simulink model "lab4_simulink3model2"  (R2024a)
settings: Solver=VariableStepAuto  StartTime=0.0  StopTime=1  RelTol=1e-3
libraries: commanabbnd3 x2
settings Model: Creator=PULLEY  LastModifiedBy=PULLEY

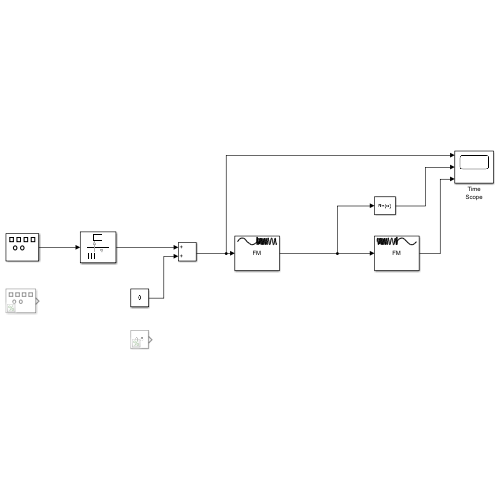
[thumbnail: Simulink's stored preview of the top-level diagram]
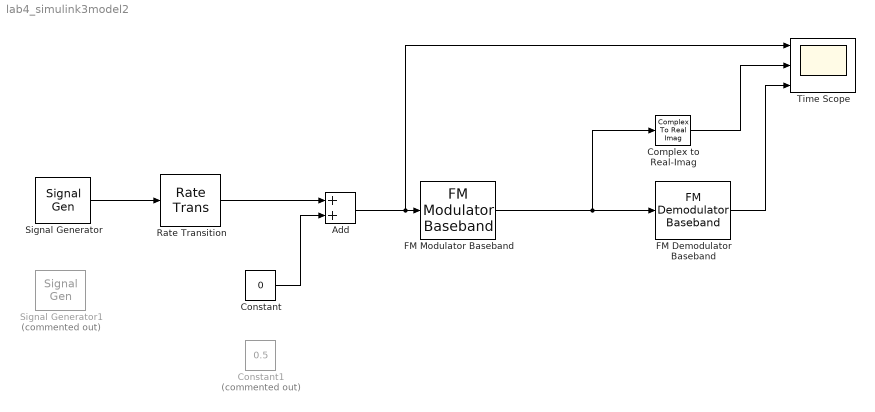
== system lab4_simulink3model2 ==
  Add : Sum
  Complex to Real-Imag : ComplexToRealImag  Output=Real
  Constant : Constant  Value=0
  Constant1 : Constant  Commented=on  Value=0.5
  "FM Demodulator Baseband " : commanabbnd3/FM Demodulator Baseband   FrequencyDeviation=100  SimulateUsing=Code generation
  FM Modulator Baseband : commanabbnd3/FM Modulator Baseband  FrequencyDeviation=100  SimulateUsing=Code generation
  Rate Transition : RateTransition  OutPortSampleTime=1/100e3
  Signal Generator : SignalGenerator  Frequency=5
  Signal Generator1 : SignalGenerator  Commented=on  WaveForm=square  Amplitude=0.5  Frequency=5
  Time Scope : Scope  NumInputPorts=3
  wires:
  Rate Transition/1 -> Add/1
  Signal Generator/1 -> Rate Transition/1
  Constant/1 -> Add/2
  Add/1 -> Time Scope/1, FM Modulator Baseband/1
  FM Modulator Baseband/1 -> "FM Demodulator Baseband "/1, Complex to Real-Imag/1
  Complex to Real-Imag/1 -> Time Scope/2
  "FM Demodulator Baseband "/1 -> Time Scope/3
